simulink model "PID_Controller"  (R2020a)
settings: Solver=VariableStepAuto  StartTime=0.0  StopTime=120.0  RelTol=1e-3
PostLoadFcn:
  | m=1000;
  | b=50;
  | u=500;
model workspace (MAT data in the model file):
  Kd = 10
  Ki = 39.43
  Kp = 847
settings Model: DataDictionary=DataDictionary.sldd  Creator=Hp  LastModifiedBy=Hp
settings DataIOCC: SaveOutput=off  SaveTime=off

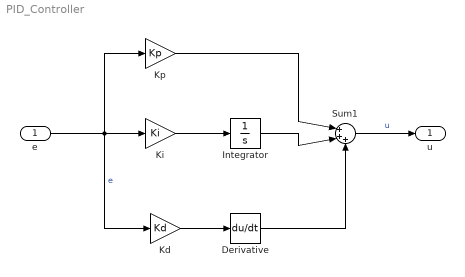
== system PID_Controller ==
  e : Inport  OutDataTypeStr=double  PortDimensions=1  SampleTime=0
  Derivative : Derivative
  Integrator : Integrator
  Kd : Gain  Gain=Kd
  Ki : Gain  Gain=Ki
  Kp : Gain  Gain=Kp
  Sum1 : Sum  Inputs=|+++
  u : Outport  OutDataTypeStr=double  PortDimensions=1  SampleTime=0
  wires:
  Integrator/1 -> Sum1/2
  Kp/1 -> Sum1/1
  Ki/1 -> Integrator/1
  e/1 -> Ki/1, Kp/1, Kd/1  "e"
  Kd/1 -> Derivative/1
  Derivative/1 -> Sum1/3
  Sum1/1 -> u/1  "u"
